simulink model "MBD_Variables_and_Model_Explorer"  (R2021b)
settings: Solver=FixedStepDiscrete  StartTime=0.0  StopTime=10.0  FixedStep=0.001  RelTol=1e-3
model workspace (MAT data in the model file):
  Noso = Simulink.Parameter
  Noso.Value = 3
  Noso.DataType = 'uint8'
  Noso.Min = 0
  Noso.Max = 5
  Noso.Complexity = 'real'
  Noso.Dimensions = [1 1]
  Param = Simulink.Parameter
  Param.DataType = 'auto'
  Param.Complexity = 'real'
  Param.Dimensions = [0 0]
  Param1 = Simulink.Parameter
  Param1.DataType = 'auto'
  Param1.Complexity = 'real'
  Param1.Dimensions = [0 0]
  Param2 = Simulink.Parameter
  Param2.DataType = 'auto'
  Param2.Complexity = 'real'
  Param2.Dimensions = [0 0]
  Param3 = Simulink.Parameter
  Param3.DataType = 'auto'
  Param3.Complexity = 'real'
  Param3.Dimensions = [0 0]
  Param4 = Simulink.Parameter
  Param4.DataType = 'auto'
  Param4.Complexity = 'real'
  Param4.Dimensions = [0 0]
values from neighbouring files (symbols this model uses):
  Noso = 5    [Model_Variables.m]
settings Model: Creator=waleed.elshemy  LastModifiedBy=waleed.elshemy

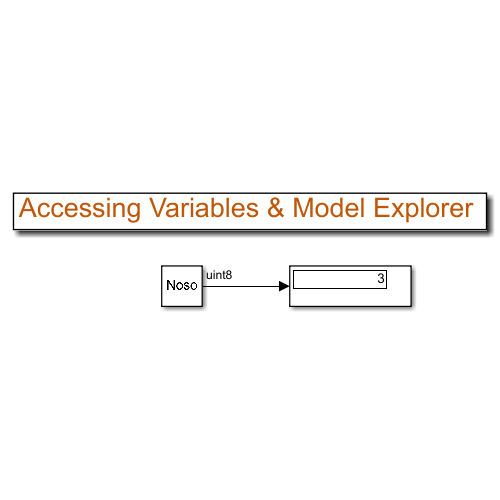
[thumbnail: Simulink's stored preview of the top-level diagram]
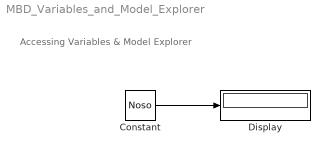
== system MBD_Variables_and_Model_Explorer ==
  note: Accessing Variables & Model Explorer
  Constant : Constant  Value=Noso
  Display : Display
  wires:
  Constant/1 -> Display/1
